simulink model "untitled5"  (R2023b)
settings: Solver=VariableStepAuto  StartTime=0.0  StopTime=0.5  RelTol=1e-3
undefined symbols (not defined in the file): D1, Delta
libraries: spsRMSLib x3, simulink_extras x3, spsThreePhaseVIMeasurementLib x2, spsThreePhaseBreakerLib x1, spsThreePhaseSeriesRLCLoadLib x1, spsThreePhaseFaultLib x1, spsThreePhaseSourceLib x1, spsThreePhaseTransformerTwoWindingsLib x1, sps_lib x1
settings Model: Creator=HP  LastModifiedBy=HP

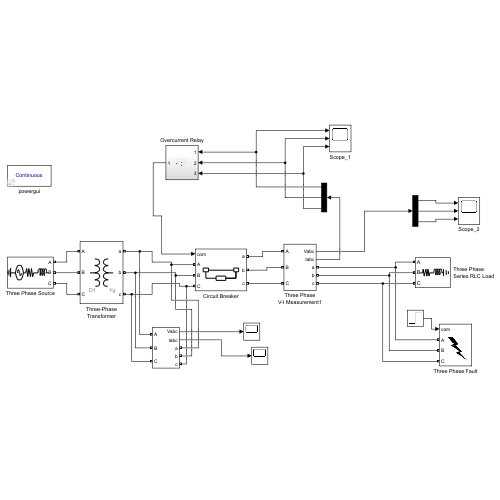
[thumbnail: Simulink's stored preview of the top-level diagram]
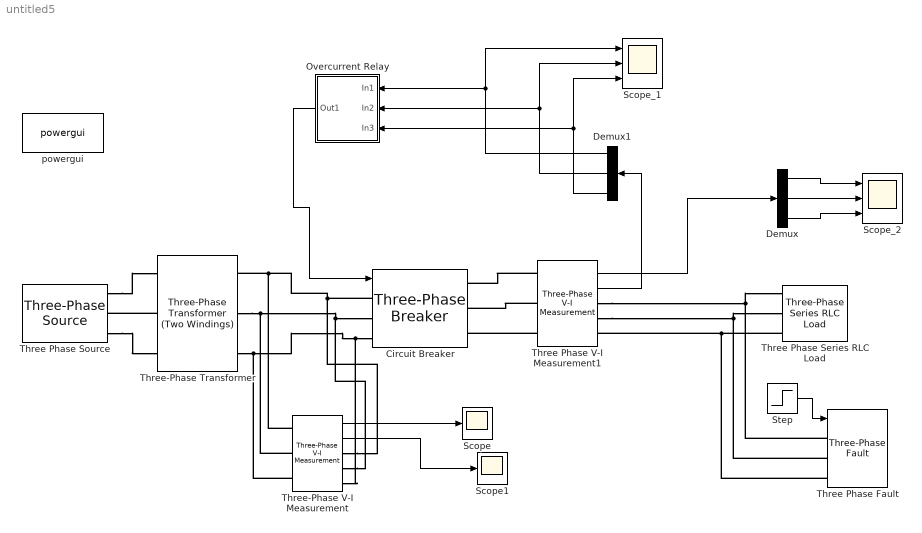
== system untitled5 ==
  Circuit Breaker : spsThreePhaseBreakerLib/Three-Phase Breaker  InitialState=closed  SwitchA=on  SwitchB=on  SwitchC=on  SwitchTimes="[1/60  5/60]"  External=on  BreakerResistance=0.01  SnubberResistance=1e6  SnubberCapacitance=inf  Measurements=None
  Demux : Demux  Outputs=3
  Demux1 : Demux  Outputs=3
  Overcurrent Relay : Subsystem
  Scope : Scope
  Scope1 : Scope
  Scope_1 : Scope  NumInputPorts=3
  Scope_2 : Scope  NumInputPorts=3
  Step : Step  Time=0.2  After=0.5  SampleTime=0
  Three Phase Series RLC Load : spsThreePhaseSeriesRLCLoadLib/Three-Phase Series RLC Load  LConnTagsString=A|B|C  Configuration=Y (grounded)  NominalVoltage=0.4e3  Vabc=[1e3 1e3 1e3]  Vabcp=[1e3 1e3 1e3]  NominalFrequency=50  UnbalancedPower=off  ActivePower=5e6  InductivePower=20e3  CapacitivePower=0  Pabc=[10e3 9e3 11e3]  QLabc=[100 90 110]  QCabc=[100 90 110]  Pabcp=[10e3 9e3 11e3]  QLabcp=[100 90 110]  QCabcp=[100 90 110]  Measurements=None  LoadType=constant Z
  Three Phase V-I Measurement1 : spsThreePhaseVIMeasurementLib/Three-Phase V-I Measurement  VoltageMeasurement=phase-to-ground  SetLabelV=off  LabelV=Vabc  Vpu=off  VpuLL=off  CurrentMeasurement=yes  SetLabelI=off  LabelI=Iabc  Ipu=off  Pbase=100e6  Vbase=500e3  OutputType=Complex  PhasorSimulation=off  PSBequivalent=0
  Three Phase Fault : spsThreePhaseFaultLib/Three-Phase Fault  InitialStates=[0 0 0]  FaultA=on  FaultB=off  FaultC=off  GroundFault=on  SwitchTimes="[1/60  5/60]"  External=on  SwitchStatus=NaN  FaultResistance=0.001  GroundResistance=0.01  SnubberResistance=1e6  SnubberCapacitance=inf  Measurements=None
  Three Phase Source : spsThreePhaseSourceLib/Three-Phase Source  InternalConnection=Yg  VoltagePhases=off  Voltage=11e3  PhaseAngle=0  Voltage_phases=[25e3 25e3 25e3]/sqrt(3)  PhaseAngles_phases=[0 -120 +120]  Frequency=50  NonIdealSource=on  SpecifyImpedance=on  Resistance=0.8929  Inductance=16.58e-3  ShortCircuitLevel=20e6  BaseVoltage=11e3  XRratio=7  BusType=swing  Pref=10e3  Qref=0  Prefabc=[10e3, 10e3, 10e3]  Qrefabc=[0, 0, 0]  Qmin=-inf  Qmax=inf
  Three-Phase Transformer : spsThreePhaseTransformerTwoWindingsLib/Three-Phase Transformer (Two Windings)  Winding1Connection=Delta (D1)  Winding2Connection=Yg  CoreType=Three single-phase transformers  SetSaturation=off  Hysteresis=off  DataFile='hysteresis'  SetInitialFlux=off  Measurements=None  UNITS=pu  NominalPower=[ 10e6 , 50 ]  Winding1=[ 11e3 , 0.002 , 0.08 ]  Winding2=[ 0.4e3 , 0.002 , 0.08 ]  Rm=500  Lm=500  L0=0.5  Saturation=[ 0,0 ; 0.0024,1.2 ; 1.0,1.52 ]  InitialFluxes=[ 0.8 , -0.8 , 0.7 ]  BreakLoop=off  DiscreteSolver=Trapezoidal iterative  DataType=off  TransfoNumber=1
  Three-Phase V-I Measurement : spsThreePhaseVIMeasurementLib/Three-Phase V-I Measurement  VoltageMeasurement=phase-to-ground  SetLabelV=off  LabelV=Vabc  Vpu=off  VpuLL=off  CurrentMeasurement=yes  SetLabelI=off  LabelI=Iabc  Ipu=off  Pbase=100e6  Vbase=500e3  OutputType=Complex  PhasorSimulation=off  PSBequivalent=0
  powergui : sps_lib/powergui  Priority=1  SimulationMode=Continuous  SampleTime=50e-6  frequency=60  Iterations=50  frequencyindice=50  Pbase=100e6  ErrMax=1e-4  UnitsV=kV  UnitsW=MW  buscounter=0  FunctionMessages=off  echomessages=off  EnableUseOfTLC=off  CurrentSourceSwitches=off  DisableSnubberDevices=off  DisableRonSwitches=off  DisableVfSwitches=off  DisplayEquations=off  AutomaticDiscreteSolvers=off  SolverType=Tustin/Backward Euler (TBE)  Interpol=off  ExternalGateDelay=off  methode=off  Ts=100  x0status=blocks  SPID=on  SwTol=0  HookPort=off  NonlinearTolerance=1e-4  nMaxIteration=100  ContinueOnMaxIteration=off  RestoreLinks=warning  ResistiveCurrentMeasurement=off  Frange=[0:2:500]  Ylog=off  Xlog=on  ShowGrid=off  save=off  variable=ZData  structure=0  ZoomFFT=off  StartTime=0.0  cycles=1  DisplayStyle=1  fundamental=60  FreqAxis=off  MaxFrequency=1000  frequencyindicesteady=1  RmsSteady=1  display=off
  wires:
  Step/1 -> Three Phase Fault/1
  Demux/1 -> Scope_2/1
  Demux/2 -> Scope_2/2
  Demux/3 -> Scope_2/3
  Three Phase V-I Measurement1/1 -> Demux/1
  Three Phase V-I Measurement1/2 -> Demux1/1
  Overcurrent Relay/1(Out1) -> Circuit Breaker/1
  Demux1/1 -> Scope_1/1, Overcurrent Relay/1(In1)
  Demux1/2 -> Scope_1/2, Overcurrent Relay/2(In2)
  Demux1/3 -> Scope_1/3, Overcurrent Relay/3(In3)
  Three-Phase V-I Measurement/1 -> Scope/1
  Three-Phase V-I Measurement/2 -> Scope1/1
  connections:
  Circuit Breaker/LConn1 -- Three-Phase V-I Measurement/LConn1 -- Three-Phase Transformer/RConn1 -- Three-Phase V-I Measurement/RConn1
  Three-Phase Transformer/RConn2 -- Three-Phase V-I Measurement/LConn2 -- Three-Phase V-I Measurement/RConn2 -- Circuit Breaker/LConn2
  Three-Phase Transformer/RConn3 -- Three-Phase V-I Measurement/LConn3 -- Three-Phase V-I Measurement/RConn3 -- Circuit Breaker/LConn3
  Three Phase V-I Measurement1/LConn1 -- Circuit Breaker/RConn1
  Three Phase V-I Measurement1/LConn2 -- Circuit Breaker/RConn2
  Three Phase V-I Measurement1/LConn3 -- Circuit Breaker/RConn3
  Three Phase Series RLC Load/LConn3 -- Three Phase Fault/LConn3 -- Three Phase V-I Measurement1/RConn3
  Three Phase V-I Measurement1/RConn2 -- Three Phase Fault/LConn2 -- Three Phase Series RLC Load/LConn2
  Three Phase V-I Measurement1/RConn1 -- Three Phase Fault/LConn1 -- Three Phase Series RLC Load/LConn1
  Three-Phase Transformer/LConn2 -- Three Phase Source/RConn2
  Three Phase Source/RConn1 -- Three-Phase Transformer/LConn1
  Three Phase Source/RConn3 -- Three-Phase Transformer/LConn3

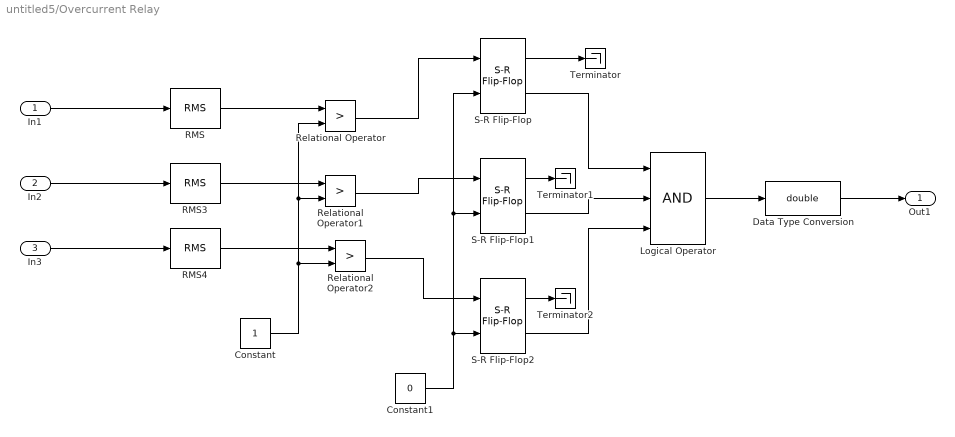
== system untitled5/Overcurrent Relay ==
  In1 : Inport
  In2 : Inport  Port=2
  In3 : Inport  Port=3
  Constant : Constant  OutDataTypeStr=boolean
  Constant1 : Constant  Value=0  OutDataTypeStr=boolean
  Data Type Conversion : DataTypeConversion  OutDataTypeStr=double  SaturateOnIntegerOverflow=off  RndMeth=Floor
  Logical Operator : Logic  Inputs=3  AllPortsSameDT=off  OutDataTypeStr=boolean
  RMS : spsRMSLib/RMS  TrueRMS=on  Freq=50  RMSInit=0  Ts=0.2
  RMS3 : spsRMSLib/RMS  TrueRMS=on  Freq=50  RMSInit=0  Ts=0.2
  RMS4 : spsRMSLib/RMS  TrueRMS=on  Freq=50  RMSInit=0  Ts=0.2
  Relational Operator : RelationalOperator  Operator=>  OutDataTypeStr=boolean  RndMeth=Simplest  InputSameDT=off
  Relational Operator1 : RelationalOperator  Operator=>  OutDataTypeStr=boolean  RndMeth=Simplest  InputSameDT=off
  Relational Operator2 : RelationalOperator  Operator=>  OutDataTypeStr=boolean  RndMeth=Simplest  InputSameDT=off
  S-R Flip-Flop : simulink_extras/Flip Flops/S-R Flip-Flop  initial_condition=0
  S-R Flip-Flop1 : simulink_extras/Flip Flops/S-R Flip-Flop  initial_condition=0
  S-R Flip-Flop2 : simulink_extras/Flip Flops/S-R Flip-Flop  initial_condition=0
  Terminator : Terminator
  Terminator1 : Terminator
  Terminator2 : Terminator
  Out1 : Outport
  wires:
  In1/1 -> RMS/1
  In3/1 -> RMS4/1
  RMS3/1 -> Relational Operator1/1
  Logical Operator/1 -> Data Type Conversion/1
  Data Type Conversion/1 -> Out1/1
  Constant1/1 -> S-R Flip-Flop2/2, S-R Flip-Flop1/2, S-R Flip-Flop/2
  Relational Operator2/1 -> S-R Flip-Flop2/1
  In2/1 -> RMS3/1
  S-R Flip-Flop/2 -> Logical Operator/1
  Constant/1 -> Relational Operator/2, Relational Operator1/2, Relational Operator2/2
  S-R Flip-Flop1/1 -> Terminator1/1
  RMS/1 -> Relational Operator/1
  Relational Operator1/1 -> S-R Flip-Flop1/1
  Relational Operator/1 -> S-R Flip-Flop/1
  RMS4/1 -> Relational Operator2/1
  S-R Flip-Flop2/2 -> Logical Operator/3
  S-R Flip-Flop2/1 -> Terminator2/1
  S-R Flip-Flop/1 -> Terminator/1
  S-R Flip-Flop1/2 -> Logical Operator/2
